simulink model "Simulationsmodell_Elektro"  (R2020b)
settings: Solver=FixedStepAuto  StartTime=0.0  StopTime=2750  FixedStep=1  RelTol=1e-3
undefined symbols (not defined in the file): c_d, c_r, eta_getriebe, fzBreite, fzBreiteInklSpiegel, fzHoehe, g, i_getriebe, i_mainreducer, kennfeld, lambda, luftdruck, M_bus, M_fahrgast, podesthoehe, R_Reifen, taupunkt, temperatur
settings Model: OrderedModelArguments=off  Creator=igyun  LastModifiedBy=zf

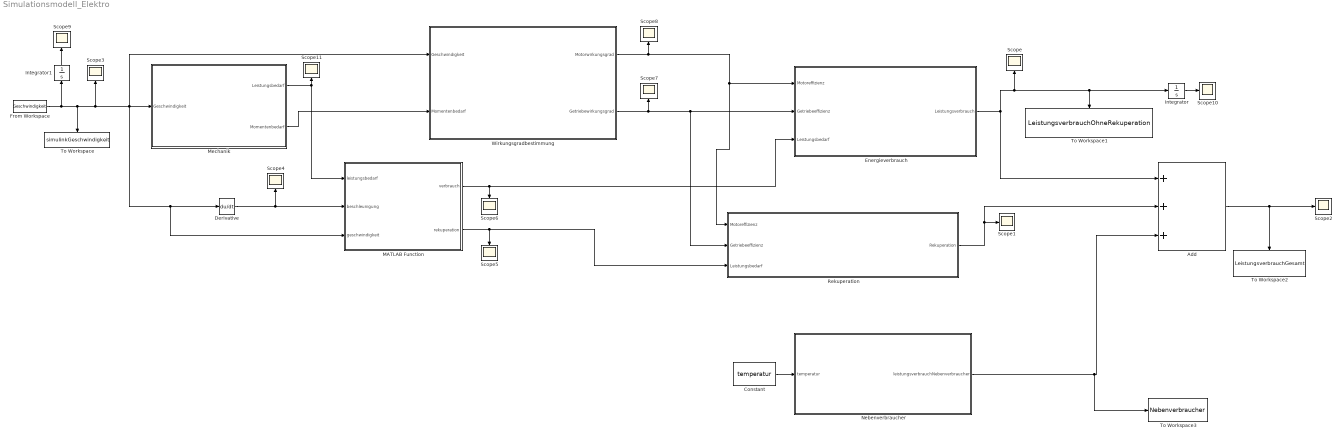
== system Simulationsmodell_Elektro ==
  Add : Sum  Inputs=+++
  Constant : Constant  Value=temperatur
  Derivative : Derivative
  Energieverbrauch : Subsystem
  From Workspace : FromWorkspace  VariableName=Geschwindigkeit
  Integrator : Integrator
  Integrator1 : Integrator
  MATLAB Function : MATLAB Function  TreatAsAtomicUnit=on
  Mechanik : Subsystem
  Nebenverbraucher : MATLAB Function  TreatAsAtomicUnit=on
  Rekuperation : Subsystem
  Scope{,1..11} (12 alike) : Scope
  To Workspace : ToWorkspace  VariableName=simulinkGeschwindigkeit  SaveFormat=Timeseries  SampleTime=-1
  To Workspace1 : ToWorkspace  VariableName=LeistungsverbrauchOhneRekuperation  SaveFormat=Timeseries  SampleTime=-1
  To Workspace2 : ToWorkspace  VariableName=LeistungsverbrauchGesamt  SaveFormat=Timeseries  SampleTime=-1
  To Workspace3 : ToWorkspace  VariableName=Nebenverbraucher  SaveFormat=Timeseries  SampleTime=-1
  Wirkungsgradbestimmung : Subsystem
  wires:
  From Workspace/1 -> Mechanik/1(Geschwindigkeit), MATLAB Function/3(geschwindigkeit), Derivative/1, Wirkungsgradbestimmung/1(Geschwindigkeit), Scope3/1, To Workspace/1, Integrator1/1
  Mechanik/2(Momentenbedarf) -> Wirkungsgradbestimmung/2(Momentenbedarf)
  Energieverbrauch/1(Leistungsverbrauch) -> Integrator/1, To Workspace1/1, Scope/1, Add/1
  Integrator1/1 -> Scope9/1
  Wirkungsgradbestimmung/2(Getriebewirkungsgrad) -> Rekuperation/2(Getriebeeffizienz), Energieverbrauch/2(Getriebeeffizienz), Scope7/1
  Wirkungsgradbestimmung/1(Motorwirkungsgrad) -> Rekuperation/1(Motoreffizienz), Energieverbrauch/1(Motoreffizienz), Scope8/1
  Mechanik/1(Leistungsbedarf) -> MATLAB Function/1(leistungsbedarf), Scope11/1
  Derivative/1 -> Scope4/1, MATLAB Function/2(beschleunigung)
  MATLAB Function/1(verbrauch) -> Energieverbrauch/3(Leistungsbedarf), Scope6/1
  MATLAB Function/2(rekuperation) -> Rekuperation/3(Leistungsbedarf), Scope5/1
  Rekuperation/1(Rekuperation) -> Scope1/1, Add/2
  Add/1 -> Scope2/1, To Workspace2/1
  Integrator/1 -> Scope10/1
  Nebenverbraucher/1(leistungsverbrauchNebenverbraucher) -> To Workspace3/1, Add/3
  Constant/1 -> Nebenverbraucher/1(temperatur)

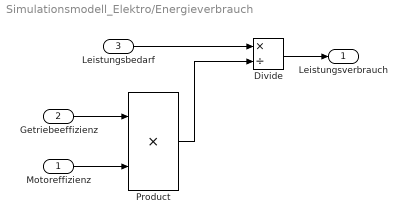
== system Simulationsmodell_Elektro/Energieverbrauch ==
  Motoreffizienz : Inport
  Getriebeeffizienz : Inport  Port=2
  Leistungsbedarf : Inport  Port=3
  Divide : Product  Inputs=*/
  Product : Product
  Leistungsverbrauch : Outport
  wires:
  Getriebeeffizienz/1 -> Product/1
  Motoreffizienz/1 -> Product/2
  Leistungsbedarf/1 -> Divide/1
  Product/1 -> Divide/2
  Divide/1 -> Leistungsverbrauch/1

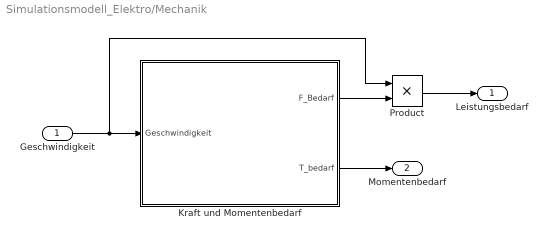
== system Simulationsmodell_Elektro/Mechanik ==
  Geschwindigkeit : Inport
  Kraft und Momentenbedarf : Subsystem
  Product : Product
  Leistungsbedarf : Outport
  Momentenbedarf : Outport  Port=2
  wires:
  Product/1 -> Leistungsbedarf/1
  Kraft und Momentenbedarf/1(F_Bedarf) -> Product/2
  Geschwindigkeit/1 -> Kraft und Momentenbedarf/1(Geschwindigkeit), Product/1
  Kraft und Momentenbedarf/2(T_bedarf) -> Momentenbedarf/1

== system Simulationsmodell_Elektro/Rekuperation ==
  Motoreffizienz : Inport
  Getriebeeffizienz : Inport  Port=2
  Leistungsbedarf : Inport  Port=3
  Product : Product  Inputs=3
  Rekuperation : Outport
  wires:
  Product/1 -> Rekuperation/1
  Leistungsbedarf/1 -> Product/1
  Motoreffizienz/1 -> Product/3
  Getriebeeffizienz/1 -> Product/2

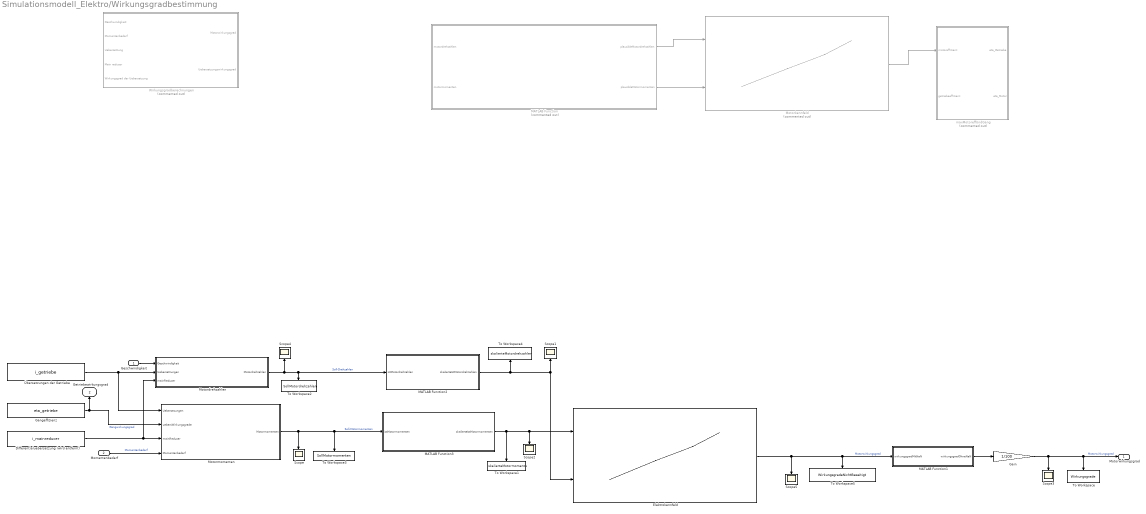
== system Simulationsmodell_Elektro/Wirkungsgradbestimmung ==
  Geschwindigkeit : Inport
  Momentenbedarf : Inport  Port=2
  Differentialuebersetzung (wird entfernt) : Constant  Value=i_mainreducer
  Elektrokennfeld : Lookup_n-D  BreakpointsForDimension1=[1:161]  BreakpointsForDimension2=[1:251]  Table=kennfeld  InterpMethod=Nearest  UseLastTableValue=on  InternalRulePriority=Speed  RndMeth=Simplest  InputSameDT=on
      settings: InputPortMap=u0,u1
  Gain : Gain  Gain=1/100
  Gangeffizienz : Constant  Value=eta_getriebe
  MATLAB Function : MATLAB Function  Commented=on  TreatAsAtomicUnit=on
  MATLAB Function1 : MATLAB Function  TreatAsAtomicUnit=on
  MATLAB Function2 : MATLAB Function  TreatAsAtomicUnit=on
  MATLAB Function3 : MATLAB Function  TreatAsAtomicUnit=on
  Motordrehzahlen : Subsystem
  Motorkennfeld : Lookup_n-D  Commented=on  BreakpointsForDimension1=[1:86]  BreakpointsForDimension2=[1:251]  Table=kennfeld  InternalRulePriority=Speed  RndMeth=Simplest  InputSameDT=on
      settings: InputPortMap=u0,u1
  Motormomenten : Subsystem
  Scope{,1..5} (6 alike) : Scope
  To Workspace : ToWorkspace  VariableName=Wirkungsgrade  SaveFormat=Timeseries  SampleTime=-1
  To Workspace1 : ToWorkspace  VariableName=skalierteMotormomente  SaveFormat=Timeseries  SampleTime=-1
  To Workspace2 : ToWorkspace  VariableName=SollMotordrehzahlen  SaveFormat=Timeseries  SampleTime=-1
  To Workspace3 : ToWorkspace  VariableName=SollMotormomenten  SaveFormat=Timeseries  SampleTime=-1
  To Workspace4 : ToWorkspace  VariableName=skalierteMotordrehzahlen  SaveFormat=Timeseries  SampleTime=-1
  To Workspace5 : ToWorkspace  VariableName=WirkungsgradeNichtBeseitigt  SaveFormat=Timeseries  SampleTime=-1
  Wirkungsgradberechnungen : Subsystem  Commented=on  TreatAsAtomicUnit=on
  maxMotoreffUndGang : MATLAB Function  Commented=on  TreatAsAtomicUnit=on
  Übersetzungen der Getriebe : Constant  Value=i_getriebe
  Motorwirkungsgrad : Outport
  Getriebewirkungsgrad : Outport  Port=2
  wires:
  Übersetzungen der Getriebe/1 -> Motormomenten/1(Uebersezungen), Motordrehzahlen/2(Uebersetzungen)
  Differentialuebersetzung (wird entfernt)/1 -> Motordrehzahlen/3(mainReducer), Motormomenten/3(mainReducer)
  Momentenbedarf/1 -> Motormomenten/4(Momentenbedarf)  "Momentenbedarf"
  MATLAB Function/1(plausibleMotordrehzahlen) -> Motorkennfeld/1
  MATLAB Function/2(plausibleMotormomenten) -> Motorkennfeld/2
  Motorkennfeld/1 -> maxMotoreffUndGang/1(motoreffizienz)
  Motordrehzahlen/1(Motordrehzahlen) -> MATLAB Function2/1(istMotordrehzahlen), To Workspace2/1, Scope4/1  "Soll-Drehzahlen"
  Motormomenten/1(Motormomenten) -> Scope/1, MATLAB Function3/1(istMotormomenten), To Workspace3/1  "Soll-Motormomenten"
  Gangeffizienz/1 -> Motormomenten/2(uebersWirkungsgrade), Getriebewirkungsgrad/1  "Gangwirkungsgrad"
  Gain/1 -> Motorwirkungsgrad/1, To Workspace/1, Scope3/1  "Motorwirkungsgrad"
  Geschwindigkeit/1 -> Motordrehzahlen/1(Geschwindigkeit)
  MATLAB Function2/1(skalierteIstMotordrehzahlen) -> Elektrokennfeld/2, Scope1/1, To Workspace4/1
  MATLAB Function3/1(skalierteIstMotormomenten) -> Elektrokennfeld/1, Scope2/1, To Workspace1/1
  Elektrokennfeld/1 -> To Workspace5/1, MATLAB Function1/1(wirkungsgradMitNaN), Scope5/1  "Motorwirkungsgrad"
  MATLAB Function1/1(wirkungsgradOhneNaN) -> Gain/1

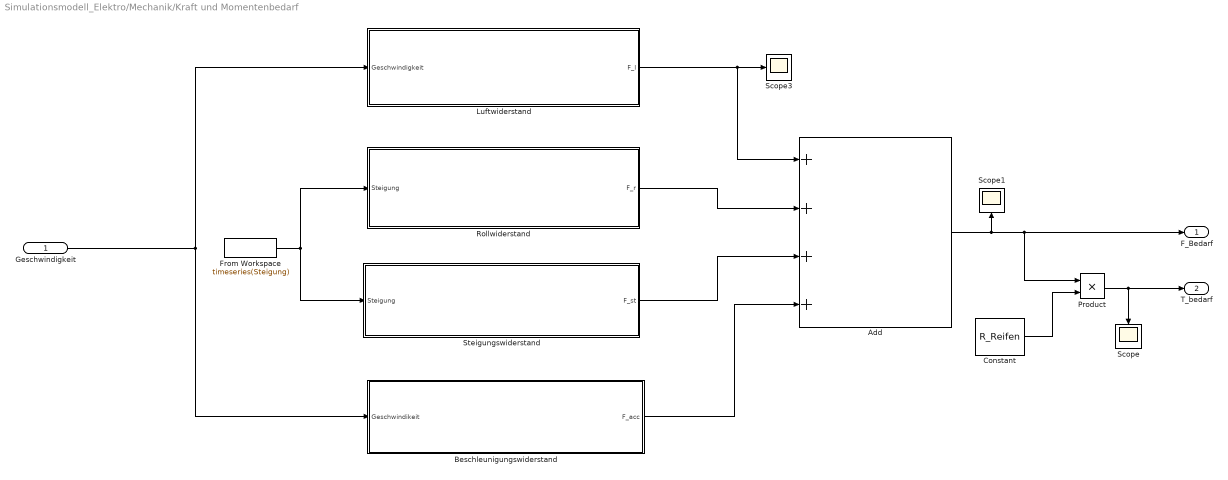
== system Simulationsmodell_Elektro/Mechanik/Kraft und Momentenbedarf ==
  Geschwindigkeit : Inport
  Add : Sum  Inputs=++++
  Beschleunigungswiderstand : Subsystem
  Constant : Constant  Value=R_Reifen
  From Workspace : FromWorkspace  VariableName=timeseries(Steigung)
  Luftwiderstand : Subsystem
  Product : Product
  Rollwiderstand : Subsystem
  Scope : Scope
  Scope1 : Scope
  Scope3 : Scope
  Steigungswiderstand : Subsystem
  F_Bedarf : Outport
  T_bedarf : Outport  Port=2
  wires:
  Geschwindigkeit/1 -> Luftwiderstand/1(Geschwindigkeit), Beschleunigungswiderstand/1(Geschwindikeit)
  Luftwiderstand/1(F_l) -> Scope3/1, Add/1
  Beschleunigungswiderstand/1(F_acc) -> Add/4
  Rollwiderstand/1(F_r) -> Add/2
  Steigungswiderstand/1(F_st) -> Add/3
  Constant/1 -> Product/2
  Product/1 -> T_bedarf/1, Scope/1
  From Workspace/1 -> Steigungswiderstand/1(Steigung), Rollwiderstand/1(Steigung)
  Add/1 -> F_Bedarf/1, Product/1, Scope1/1

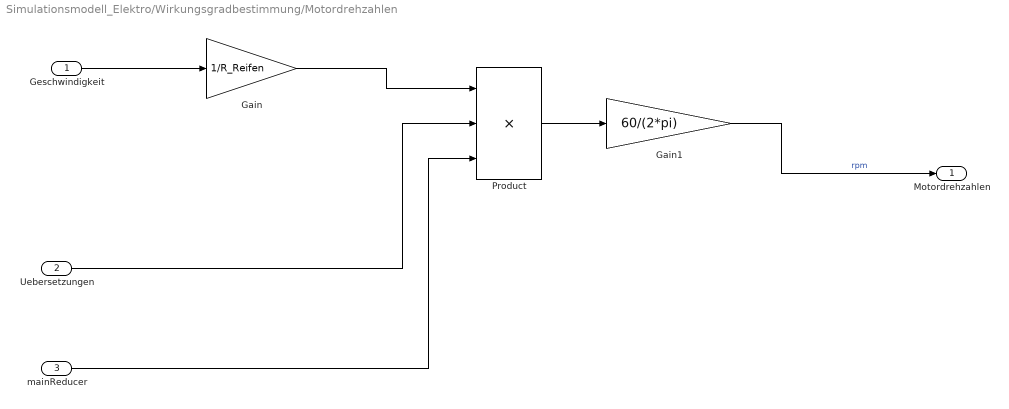
== system Simulationsmodell_Elektro/Wirkungsgradbestimmung/Motordrehzahlen ==
  Geschwindigkeit : Inport
  Uebersetzungen : Inport  Port=2
  mainReducer : Inport  Port=3
  Gain : Gain  Gain=1/R_Reifen
  Gain1 : Gain  Gain=60/(2*pi)
  Product : Product  Inputs=3
  Motordrehzahlen : Outport
  wires:
  Geschwindigkeit/1 -> Gain/1
  Product/1 -> Gain1/1
  Uebersetzungen/1 -> Product/2
  Gain/1 -> Product/1
  mainReducer/1 -> Product/3
  Gain1/1 -> Motordrehzahlen/1  "rpm"

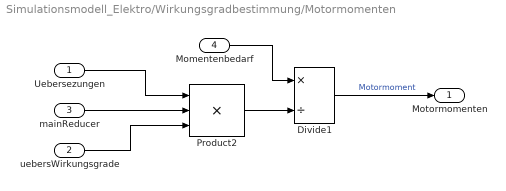
== system Simulationsmodell_Elektro/Wirkungsgradbestimmung/Motormomenten ==
  Uebersezungen : Inport
  uebersWirkungsgrade : Inport  Port=2
  mainReducer : Inport  Port=3
  Momentenbedarf : Inport  Port=4
  Divide1 : Product  Inputs=*/
  Product2 : Product  Inputs=3
  Motormomenten : Outport
  wires:
  uebersWirkungsgrade/1 -> Product2/3
  mainReducer/1 -> Product2/2
  Product2/1 -> Divide1/2
  Momentenbedarf/1 -> Divide1/1
  Uebersezungen/1 -> Product2/1
  Divide1/1 -> Motormomenten/1  "Motormoment"

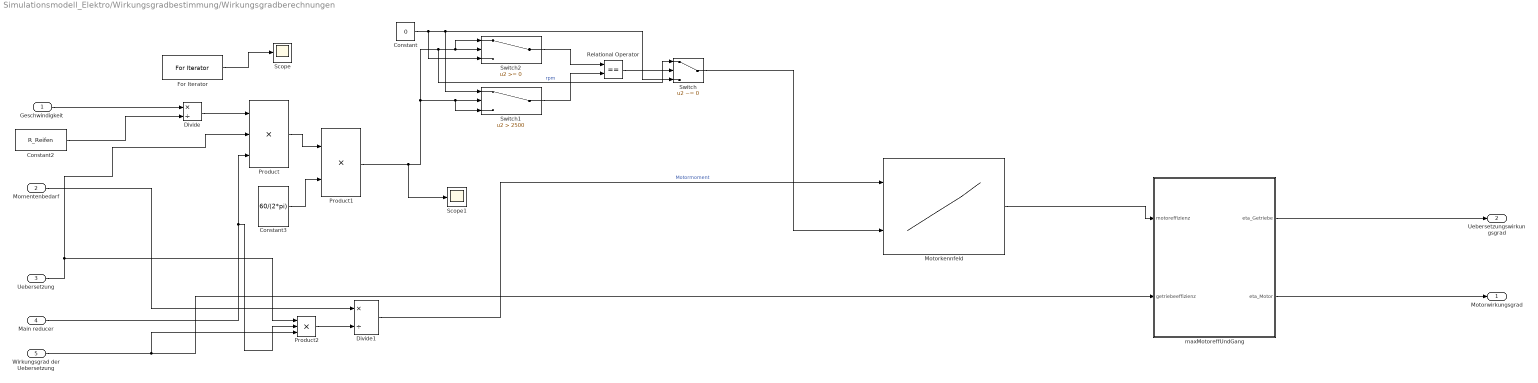
== system Simulationsmodell_Elektro/Wirkungsgradbestimmung/Wirkungsgradberechnungen ==
  Geschwindigkeit : Inport
  Momentenbedarf : Inport  Port=2
  Uebersetzung : Inport  Port=3
  Main reducer : Inport  Port=4
  Wirkungsgrad der Uebersetzung : Inport  Port=5
  Constant : Constant  Value=0
  Constant2 : Constant  Value=R_Reifen
  Constant3 : Constant  Value=60/(2*pi)
  Divide : Product  Inputs=*/
  Divide1 : Product  Inputs=*/
  For Iterator : ForIterator  IterationLimit=4
  Motorkennfeld : Lookup_n-D  BreakpointsForDimension1=[1:86]  BreakpointsForDimension2=[1:251]  Table=kennfeld  InternalRulePriority=Speed  RndMeth=Simplest  InputSameDT=on
      settings: InputPortMap=u0,u1
  Product : Product  Inputs=3
  Product1 : Product
  Product2 : Product  Inputs=3
  Relational Operator : RelationalOperator  Operator===  OutDataTypeStr=boolean  RndMeth=Simplest
  Scope : Scope
  Scope1 : Scope
  Switch : Switch  Criteria=u2 ~= 0  Threshold=1
  Switch1 : Switch  Criteria=u2 > Threshold  Threshold=2500
  Switch2 : Switch
  maxMotoreffUndGang : MATLAB Function  TreatAsAtomicUnit=on
  Motorwirkungsgrad : Outport
  Uebersetzungswirkungsgrad : Outport  Port=2
  wires:
  Constant3/1 -> Product1/2
  Product/1 -> Product1/1
  Constant2/1 -> Divide/2
  Geschwindigkeit/1 -> Divide/1
  Divide/1 -> Product/1
  Wirkungsgrad der Uebersetzung/1 -> maxMotoreffUndGang/2(getriebeeffizienz), Product2/3
  Main reducer/1 -> Product2/2, Product/3
  Uebersetzung/1 -> Product/2, Product2/1
  Product2/1 -> Divide1/2
  Momentenbedarf/1 -> Divide1/1
  Divide1/1 -> Motorkennfeld/1  "Motormoment"
  Motorkennfeld/1 -> maxMotoreffUndGang/1(motoreffizienz)
  maxMotoreffUndGang/1(eta_Getriebe) -> Uebersetzungswirkungsgrad/1
  maxMotoreffUndGang/2(eta_Motor) -> Motorwirkungsgrad/1
  For Iterator/1 -> Scope/1
  Switch2/1 -> Relational Operator/1
  Switch1/1 -> Relational Operator/2
  Constant/1 -> Switch2/3, Switch1/1, Switch/3
  Switch/1 -> Motorkennfeld/2
  Relational Operator/1 -> Switch/2
  Product1/1 -> Scope1/1, Switch1/3, Switch1/2, Switch/1, Switch2/1, Switch2/2  "rpm"

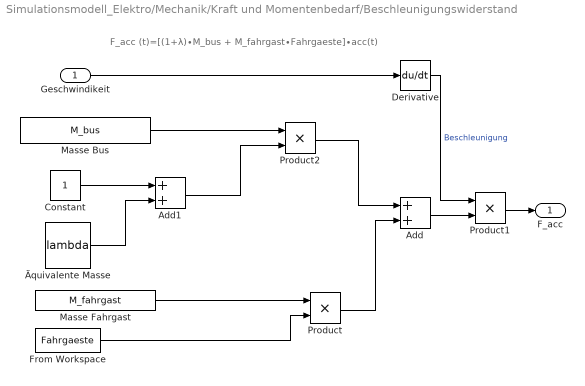
== system Simulationsmodell_Elektro/Mechanik/Kraft und Momentenbedarf/Beschleunigungswiderstand ==
  note: F_acc (t)=[(1+λ)∙M_bus + M_fahrgast∙Fahrgaeste]∙acc(t)
  Geschwindikeit : Inport
  Add : Sum
  Add1 : Sum
  Constant : Constant
  Derivative : Derivative
  From Workspace : FromWorkspace  VariableName=Fahrgaeste
  Masse Bus : Constant  Value=M_bus
  Masse Fahrgast : Constant  Value=M_fahrgast
  Product : Product
  Product1 : Product
  Product2 : Product
  Äquivalente Masse : Constant  Value=lambda
  F_acc : Outport
  wires:
  Geschwindikeit/1 -> Derivative/1
  Masse Fahrgast/1 -> Product/1
  From Workspace/1 -> Product/2
  Product/1 -> Add/2
  Constant/1 -> Add1/1
  Äquivalente Masse/1 -> Add1/2
  Derivative/1 -> Product1/1  "Beschleunigung"
  Add/1 -> Product1/2
  Product1/1 -> F_acc/1
  Product2/1 -> Add/1
  Masse Bus/1 -> Product2/1
  Add1/1 -> Product2/2

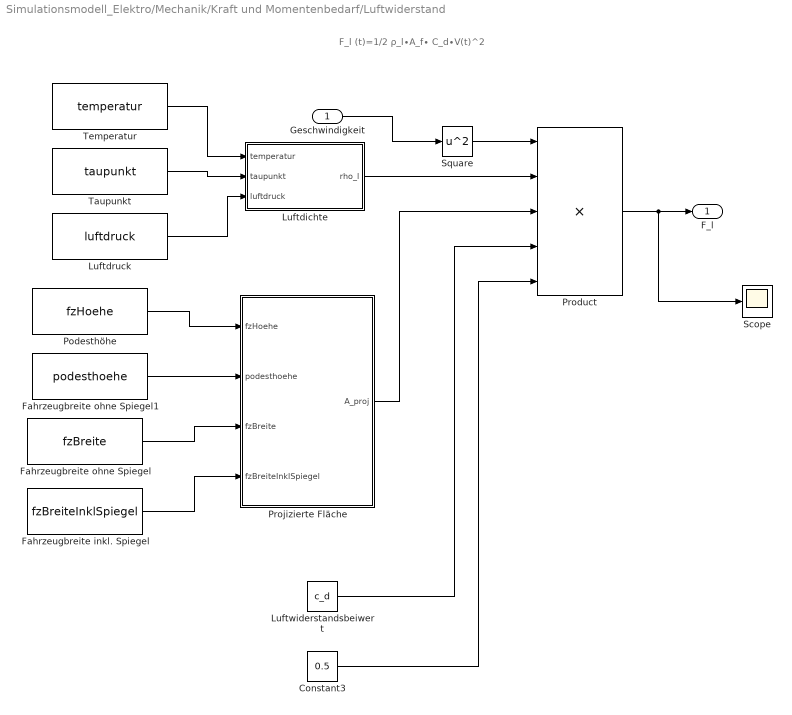
== system Simulationsmodell_Elektro/Mechanik/Kraft und Momentenbedarf/Luftwiderstand ==
  note: F_l (t)=1/2 ρ_l∙A_f∙ C_d∙V(t)^2
  Geschwindigkeit : Inport
  Constant3 : Constant  Value=0.5
  Fahrzeugbreite inkl. Spiegel : Constant  Value=fzBreiteInklSpiegel
  Fahrzeugbreite ohne Spiegel : Constant  Value=fzBreite
  Fahrzeugbreite ohne Spiegel1 : Constant  Value=podesthoehe
  Luftdichte : MATLAB Function  TreatAsAtomicUnit=on
  Luftdruck : Constant  Value=luftdruck
  Luftwiderstandsbeiwert : Constant  Value=c_d
  Podesthöhe : Constant  Value=fzHoehe
  Product : Product  Inputs=5
  Projizierte Fläche : MATLAB Function  TreatAsAtomicUnit=on
  Scope : Scope
  Square : Math  Operator=square  SaturateOnIntegerOverflow=on
  Taupunkt : Constant  Value=taupunkt
  Temperatur : Constant  Value=temperatur
  F_l : Outport
  wires:
  Geschwindigkeit/1 -> Square/1
  Square/1 -> Product/1
  Luftdichte/1(rho_l) -> Product/2
  Projizierte Fläche/1(A_proj) -> Product/3
  Luftwiderstandsbeiwert/1 -> Product/4
  Constant3/1 -> Product/5
  Product/1 -> Scope/1, F_l/1
  Temperatur/1 -> Luftdichte/1(temperatur)
  Taupunkt/1 -> Luftdichte/2(taupunkt)
  Luftdruck/1 -> Luftdichte/3(luftdruck)
  Fahrzeugbreite inkl. Spiegel/1 -> Projizierte Fläche/4(fzBreiteInklSpiegel)
  Fahrzeugbreite ohne Spiegel/1 -> Projizierte Fläche/3(fzBreite)
  Fahrzeugbreite ohne Spiegel1/1 -> Projizierte Fläche/2(podesthoehe)
  Podesthöhe/1 -> Projizierte Fläche/1(fzHoehe)

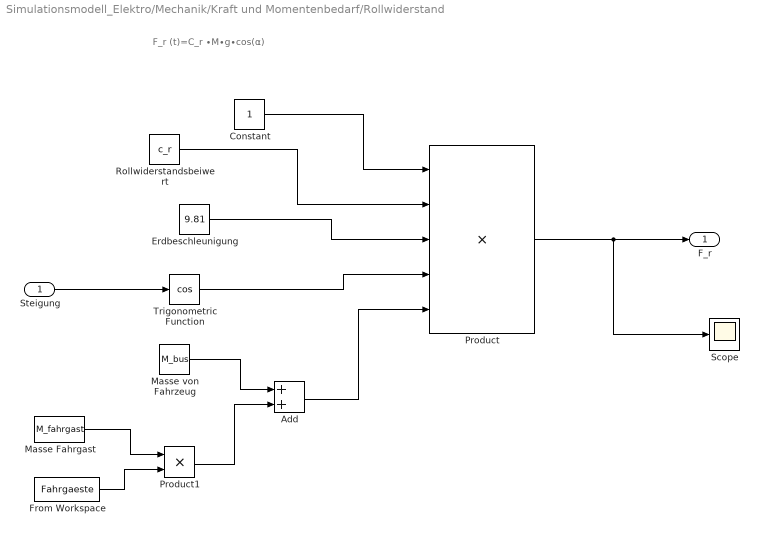
== system Simulationsmodell_Elektro/Mechanik/Kraft und Momentenbedarf/Rollwiderstand ==
  note: F_r (t)=C_r ∙M∙g∙cos⁡(α)
  Steigung : Inport
  Add : Sum
  Constant : Constant
  Erdbeschleunigung : Constant  Value=9.81
  From Workspace : FromWorkspace  VariableName=Fahrgaeste
  Masse Fahrgast : Constant  Value=M_fahrgast
  Masse von Fahrzeug : Constant  Value=M_bus
  Product : Product  Inputs=5
  Product1 : Product
  Rollwiderstandsbeiwert : Constant  Value=c_r
  Scope : Scope
  Trigonometric Function : Trigonometry  Operator=cos
  F_r : Outport
  wires:
  Masse von Fahrzeug/1 -> Add/1
  Steigung/1 -> Trigonometric Function/1
  Add/1 -> Product/5
  Trigonometric Function/1 -> Product/4
  Erdbeschleunigung/1 -> Product/3
  Rollwiderstandsbeiwert/1 -> Product/2
  Product/1 -> Scope/1, F_r/1
  Masse Fahrgast/1 -> Product1/1
  From Workspace/1 -> Product1/2
  Product1/1 -> Add/2
  Constant/1 -> Product/1

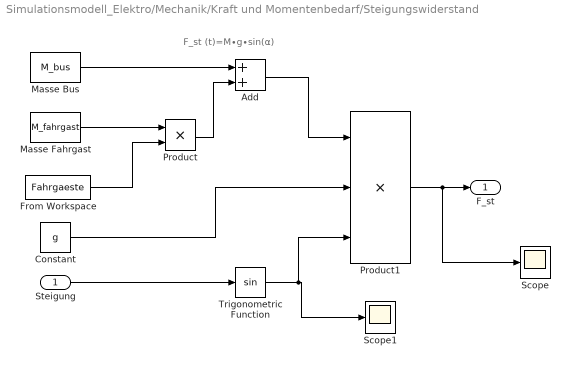
== system Simulationsmodell_Elektro/Mechanik/Kraft und Momentenbedarf/Steigungswiderstand ==
  note: F_st (t)=M∙g∙sin⁡(α)
  Steigung : Inport
  Add : Sum
  Constant : Constant  Value=g
  From Workspace : FromWorkspace  VariableName=Fahrgaeste
  Masse Bus : Constant  Value=M_bus
  Masse Fahrgast : Constant  Value=M_fahrgast
  Product : Product
  Product1 : Product  Inputs=3
  Scope : Scope
  Scope1 : Scope
  Trigonometric Function : Trigonometry
  F_st : Outport
  wires:
  Masse Fahrgast/1 -> Product/1
  From Workspace/1 -> Product/2
  Masse Bus/1 -> Add/1
  Product/1 -> Add/2
  Steigung/1 -> Trigonometric Function/1
  Add/1 -> Product1/1
  Trigonometric Function/1 -> Product1/3, Scope1/1
  Product1/1 -> Scope/1, F_st/1
  Constant/1 -> Product1/2

== matlab function Simulationsmodell_Elektro/Mechanik/Kraft und Momentenbedarf/Luftwiderstand/Projizierte Fläche ==
  data: fzHoehe input; A_proj output; podesthoehe input; fzBreite input; fzBreiteInklSpiegel input
function A_proj = projflaeche(fzHoehe, podesthoehe, fzBreite, fzBreiteInklSpiegel)

    %Eingabe in Maske: mm
    
    A_proj1 = (fzHoehe-podesthoehe)*fzBreite;
    
    %Spiegelhöhe
    spiegelHoehe = 400;
    A_proj2 = (fzBreiteInklSpiegel-fzBreite)*spiegelHoehe;
    
    A_proj = A_proj1 + A_proj2;
    
    %Umrechung mm^2 in m^2;
    
    A_proj = A_proj * 10^-6;
    
end

== matlab function Simulationsmodell_Elektro/Mechanik/Kraft und Momentenbedarf/Luftwiderstand/Luftdichte ==
  data: temperatur input; rho_l output; taupunkt input; luftdruck input
function rho_l = luftdichte(temperatur, taupunkt, luftdruck)

%Für Werte: https://kachelmannwetter.com/site/auswahl

%Einheiten bei der Eingabemaske:
%Druck: hPa
%Temperatur: Celsius

%Temperaturumrechnung
temperatur = temperatur + 273.15;



%Konstanten aus https://www.gribble.org/cycling/air_density.html
c0 = 0.99999683;
c1 = -0.90826951e-2;
c2 = 0.78736169e-4;
c3 = -0.61117958e-6;
c4 = 0.43884187e-8;
c5 = -0.29883885e-10;
c6 = 0.21874425e-12;
c7 = -0.17892321e-14;
c8 = 0.11112018e-16;
c9 = -0.30994571e-19;

e_so = 6.1078;

R_v = 461.4964;
R_d=287.0531;

%Druck bei Sättigungstemperatur
p_taupunkt = c0 + taupunkt *(c1 + taupunkt*(c2 + taupunkt*(c3 + taupunkt*(c4 + taupunkt*(c5 + taupunkt*(c6 + taupunkt*(c7 + taupunkt*(c8 + taupunkt*(c9) ) ) ) ) ) ) ));

%Sättigungsdruck von Dampf
E_s = e_so./p_taupunkt.^8;
P_v = E_s;

%Luftdruck bei trockener Luft
P_d = luftdruck - P_v;

%Luftdichte in kg/m^3
rho_l =  (P_d*100 / (R_d * temperatur)) + (P_v*100 / (R_v * temperatur));
%Umrechnungsfaktor 100 von mbar(hPa) zu Pa
end

== matlab function Simulationsmodell_Elektro/Wirkungsgradbestimmung/MATLAB Function ==
  data: motordrehzahlen input; plausibleMotordrehzahlen output; motormomenten input; plausibleMotormomenten output
function [plausibleMotordrehzahlen, plausibleMotormomenten] = ueberpruefenDrehzahlDrehmoment(motordrehzahlen, motormomenten)
    %Vorerzeugen der Vektoren mit plausiblen Daten
    plausibleMotordrehzahlen = zeros(4,1);
    plausibleMotormomenten = zeros(4,1);
    for j = 1:4 %4 Gänge => 4 drehzahlen bzw. momenten
        if motordrehzahlen(j)<=2500 && motordrehzahlen(j)>=800 && motormomenten(j)>=0 && motormomenten(j)<=1200
            %Wenn die Bedingungen erfüllt sind, ist der Betriebspunkt
            %erreichbar
            plausibleMotordrehzahlen(j,1)=motordrehzahlen(j);
            plausibleMotormomenten(j,1)=motormomenten(j);
        else
            plausibleMotordrehzahlen(j,1)=0;
            plausibleMotormomenten(j,1)=0;
        end
    end
end

== matlab function Simulationsmodell_Elektro/Wirkungsgradbestimmung/Wirkungsgradberechnungen/maxMotoreffUndGang ==
  data: motoreffizienz input; eta_Getriebe output; getriebeeffizienz input; eta_Motor output
function [eta_Getriebe, eta_Motor] = wirkungsgradAuswahl(motoreffizienz, getriebeeffizienz)

for j = 2:length(motoreffizienz)
    if motoreffizienz(j)>motoreffizienz(j-1)
        index = j;
    else
        index = j-1;
    end
end
eta_Getriebe = getriebeeffizienz(index);
eta_Motor = motoreffizienz(index);

== matlab function Simulationsmodell_Elektro/Wirkungsgradbestimmung/maxMotoreffUndGang ==
  data: motoreffizienz input; eta_Getriebe output; getriebeeffizienz input; eta_Motor output
function [eta_Getriebe, eta_Motor] = wirkungsgradAuswahl(motoreffizienz, getriebeeffizienz)

for j = 2:length(motoreffizienz)
    if motoreffizienz(j)>motoreffizienz(j-1)
        index = j;
    else
        index = j-1;
    end
end
eta_Getriebe = getriebeeffizienz(index);
eta_Motor = motoreffizienz(index);

== matlab function Simulationsmodell_Elektro/MATLAB Function ==
  data: leistungsbedarf input; verbrauch output; beschleunigung input; rekuperation output; geschwindigkeit input
function [verbrauch, rekuperation] = leistungsbedarfFallunterscheidung(leistungsbedarf, beschleunigung, geschwindigkeit)

    if leistungsbedarf > 0
        %Positiver Leistungsbedarf => Verbrauch
        verbrauch = leistungsbedarf;
        rekuperation = 0;
    else
        %Negativer Leistungsbedarf => Möglichkeit zur Rekuperation
        %Teil-Rekuperation
        if (geschwindigkeit >= 1.5 && geschwindigkeit < 3) && ( (beschleunigung<0) && (beschleunigung >= -4))
            verbrauch = 0;
            rekuperationsanteil = -1 + 2/3*geschwindigkeit;
            rekuperation = rekuperationsanteil .* leistungsbedarf;
            
        %Voll-Rekuperation
        elseif geschwindigkeit >= 3 && ((beschleunigung<0) && (beschleunigung >= -2.5))
            verbrauch = 0;
            rekuperation = leistungsbedarf;
        %Keine Rekuperation
        else
            verbrauch = 0;
            rekuperation = 0;
        end
    end


end

== matlab function Simulationsmodell_Elektro/Wirkungsgradbestimmung/MATLAB Function1 ==
  data: wirkungsgradMitNaN input; wirkungsgradOhneNaN output
function wirkungsgradOhneNaN = nanBeseitigen(wirkungsgradMitNaN)

    %Annahme: wenn kein Wert in Kennfeld vorhanden => eta = 80%

    if isnan(wirkungsgradMitNaN)
        wirkungsgradOhneNaN = 60;
    else
        wirkungsgradOhneNaN=wirkungsgradMitNaN;
    end
end

== matlab function Simulationsmodell_Elektro/Wirkungsgradbestimmung/MATLAB Function3 ==
  data: istMotormomenten input; skalierteIstMotormomenten output
function skalierteIstMotormomenten = skalierungMoment(istMotormomenten)

    %Motormomentbereich des verwendeten Kennfelds 
    %torqueBereichKennfeld = [minKennfeldTorque; maxKennfeldTorque]
    %Einheit: Nm
    %----------!!!Anpassungsbedarf!!!-----------
    minKennfeldTorque = 1;
    maxKennfeldTorque = 161;
    
    torqueBereichKennfeld = maxKennfeldTorque - minKennfeldTorque;
    
    
    %Motormomentbereich des Motors
    %torqueBereichMotor = [minMotorTorque, maxMotorTorque]
    %Einheit Nm
    minMotorTorque = -970;
    maxMotorTorque = 970;
    
    torqueBereichMotor = maxMotorTorque - minMotorTorque;
    
    %Formel
    skalierteIstMotormomenten = minKennfeldTorque + (torqueBereichKennfeld/torqueBereichMotor)*(istMotormomenten-minMotorTorque);

end

== matlab function Simulationsmodell_Elektro/Wirkungsgradbestimmung/MATLAB Function2 ==
  data: istMotordrehzahlen input; skalierteIstMotordrehzahlen output
function skalierteIstMotordrehzahlen  = skalierungDrehzahl(istMotordrehzahlen)

    %Drehzahlenbereich des verwendeten Kennfelds 
    %rpmBereichKennfeld = [minKennfeldRPM; maxKennfeldRPM]
    %Einheit: U/min
    %----------!!!Anpassungsbedarf!!!-----------
    minKennfeldRPM = 1;
    maxKennfeldRPM = 251;
    
    rpmBereichKennfeld = maxKennfeldRPM - minKennfeldRPM;
    
    
    %Drehzahlenbereich des Motors
    %rpmBereichMotor = [minMotorRPM, maxMotorRPM]
    %Einheit U/min
    minMotorRPM = 0;
    maxMotorRPM = 11000;
    
    rpmBereichMotor = maxMotorRPM - minMotorRPM;
    
    %Formel
    skalierteIstMotordrehzahlen = minKennfeldRPM + (rpmBereichKennfeld/rpmBereichMotor)*(istMotordrehzahlen-minMotorRPM);
end

== matlab function Simulationsmodell_Elektro/Nebenverbraucher ==
  data: temperatur input; leistungsverbrauchNebenverbraucher output
function leistungsverbrauchNebenverbraucher = nebenverbraucherLeistung(temperatur)


if temperatur >= 10 && temperatur <=20
    
    leistungsverbrauchNebenverbraucher = 5000;
    
elseif temperatur > 20 && temperatur <= 40
    %Annahme: 5kW bis 14kW
    %lineare Interpolation
    %leistungsverbrauchNebenverbraucher = -4000+450.*temperatur;
    tempPunkte = [20 40];
    leistPunkte = [5000 14000];
    leistungsverbrauchNebenverbraucher = interp1(tempPunkte, leistPunkte, temperatur);
    
elseif temperatur > 40
    %Annahme: 14 kW
    leistungsverbrauchNebenverbraucher = 14000;
    
elseif temperatur >= -25 && temperatur <= -10
    
    %Annahme: Linearer Verbrauch 10kW bis 15kW
    %leistungsverbrauchNebenverbraucher = 20000/3 - 1000/3 .* temperatur;
    tempPunkte = [-25 -10];
    leistPunkte = [15000 10000];
    leistungsverbrauchNebenverbraucher = interp1(tempPunkte, leistPunkte, temperatur);

elseif temperatur < 10 && temperatur > - 10
    
    %Annahme von 5kW bis 10kW
    %leistungsverbrauchNebenverbraucher = 7500-250.*temperatur;
    
    tempPunkte = [-10 10];
    leistPunkte = [10000 5000];
    leistungsverbrauchNebenverbraucher = interp1(tempPunkte, leistPunkte, temperatur);

else
    %Extreme cold
    leistungsverbrauchNebenverbraucher = 22000;
    
end
